simulink library "INT_CoVMD_SpdCoord"  (R2016b)
settings: Solver=VariableStepAuto  StartTime=0.0  StopTime=10.0  RelTol=1e-3
settings Model: Creator=Administrator  LastModifiedBy=Administrator

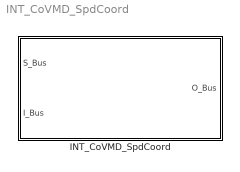
== system INT_CoVMD_SpdCoord ==
  INT_CoVMD_SpdCoord : Subsystem

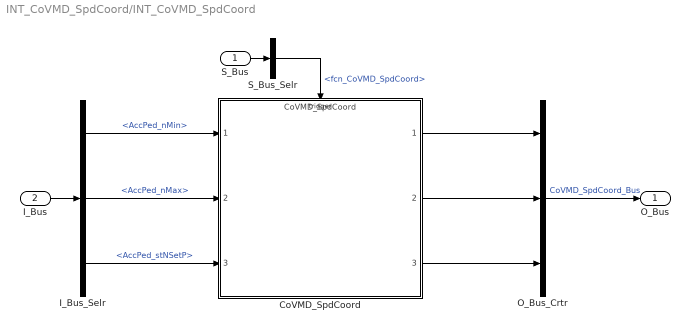
== system INT_CoVMD_SpdCoord/INT_CoVMD_SpdCoord ==
  S_Bus : Inport
  I_Bus : Inport  Port=2
  CoVMD_SpdCoord : ModelReference  ModelNameDialog=CoVMD_SpdCoord  SimulationMode=Normal  ModelReferenceVersion=1.7  TriggerPortName=function  TriggerPortTriggerType=function-call  TriggerPortStatesWhenEnabling=held
  I_Bus_Selr : BusSelector  OutputSignals=AccPed_nMin,AccPed_nMax,AccPed_stNSetP
  O_Bus_Crtr : BusCreator  Inputs=3
  S_Bus_Selr : BusSelector  OutputSignals=fcn_CoVMD_SpdCoord
  O_Bus : Outport
  wires:
  S_Bus_Selr/1 -> CoVMD_SpdCoord/Trigger  "<fcn_CoVMD_SpdCoord>"
  S_Bus/1 -> S_Bus_Selr/1
  I_Bus/1 -> I_Bus_Selr/1
  I_Bus_Selr/1 -> CoVMD_SpdCoord/1  "<AccPed_nMin>"
  I_Bus_Selr/2 -> CoVMD_SpdCoord/2  "<AccPed_nMax>"
  I_Bus_Selr/3 -> CoVMD_SpdCoord/3  "<AccPed_stNSetP>"
  O_Bus_Crtr/1 -> O_Bus/1  "CoVMD_SpdCoord_Bus"
  CoVMD_SpdCoord/1 -> O_Bus_Crtr/1
  CoVMD_SpdCoord/2 -> O_Bus_Crtr/2
  CoVMD_SpdCoord/3 -> O_Bus_Crtr/3
